simulink model "GSFR_with_P_sigIn"  (R2019b)
settings: Solver=VariableStepAuto  StartTime=0  StopTime=20.0  MaxStep=0.01  RelTol=1e-3
model workspace (MAT data in the model file):
  H = [8 1]
values from neighbouring files (symbols this model uses):
  Pd = -0.1    [Monte_Carlo_GSFR_Ideal_Injection.m]    (also in Pd_and_Injection_Model_Run.m = -0.3; Simulink_Approach_Jesus.m = -0.3; dpt_from_dft_H.m = -0.3)
settings Model: EnablePacing=on  PacingRate=1000  ParameterArgumentNames=H  OrderedModelArguments=off  Creator=ruiva  LastModifiedBy=ruiva

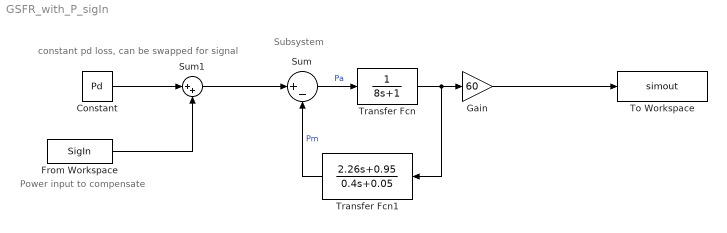
== system GSFR_with_P_sigIn ==
  note: Power input to compensate
  note: constant pd loss, can be swapped for signal
  note: Subsystem
  Constant : Constant  Value=Pd
  From Workspace : FromWorkspace  VariableName=SigIn  SampleTime=0
  Gain : Gain  Gain=60
  Sum : Sum  Inputs=|+-
  Sum1 : Sum  Inputs=|++
  To Workspace : ToWorkspace  VariableName=simout  SampleTime=-1
  Transfer Fcn : TransferFcn  Denominator=[8 1]
  Transfer Fcn1 : TransferFcn  Numerator=[2.26 0.95]  Denominator=[0.4 0.05]
  wires:
  Transfer Fcn1/1 -> Sum/2  "Pm"
  Transfer Fcn/1 -> Transfer Fcn1/1, Gain/1
  Gain/1 -> To Workspace/1
  Sum/1 -> Transfer Fcn/1  "Pa"
  Constant/1 -> Sum1/1
  Sum1/1 -> Sum/1
  From Workspace/1 -> Sum1/2
